simulink model "cesta"  (R2013a)
settings: Solver=ode3  StartTime=0.0  StopTime=10  FixedStep=0.01  RelTol=1e-3
values from neighbouring files (symbols this model uses):
  goalX = 900    [start.m]
  goalY = 900    [start.m]
  k1 = patch ([posx p1(1) p2(1) posx],[posy p1(2) p2(2) posy],'blue')    [start.m]    (also in viewMap.m = u(10))
  k2 = patch ([posx p2(1) p3(1) posx],[posy p2(2) p3(2) posy],'blue')    [start.m]    (also in viewMap.m = u(12))
  k3 = patch ([posx p3(1) p4(1) posx],[posy p3(2) p4(2) posy],'blue')    [start.m]    (also in viewMap.m = u(14))
  map = genRandMap(100,100,50)    [dummyTest.m]    (also in genRandMap.m = zeros(rows,columns); start.m)
  posx = 50    [start.m]
  posy = 50    [start.m]
  refAuto = patch([posx-xSize/2 posx+xSize/2 posx+xSize/2 posx-xSize/2], [posy-ySize/2 posy-ySize/2 posy+ySize/2 posy+ySize/2], 'green')    [start.m]    (also in viewMap.m = u(7))
  refK1 = patch ([posx p1(1) p2(1) posx],[posy p1(2) p2(2) posy],'blue')    [start.m]    (also in viewMap.m = u(9))
  refK2 = patch ([posx p2(1) p3(1) posx],[posy p2(2) p3(2) posy],'blue')    [start.m]    (also in viewMap.m = u(11))
  refK3 = patch ([posx p3(1) p4(1) posx],[posy p3(2) p4(2) posy],'blue')    [start.m]    (also in viewMap.m = u(13))
  sensRange = 100    [start.m]
undefined symbols (not defined in the file or in its folder): evalObstacles, viewMap
libraries: fuzblock x1
settings Model: Creator=Marek  LastModifiedBy=Marek

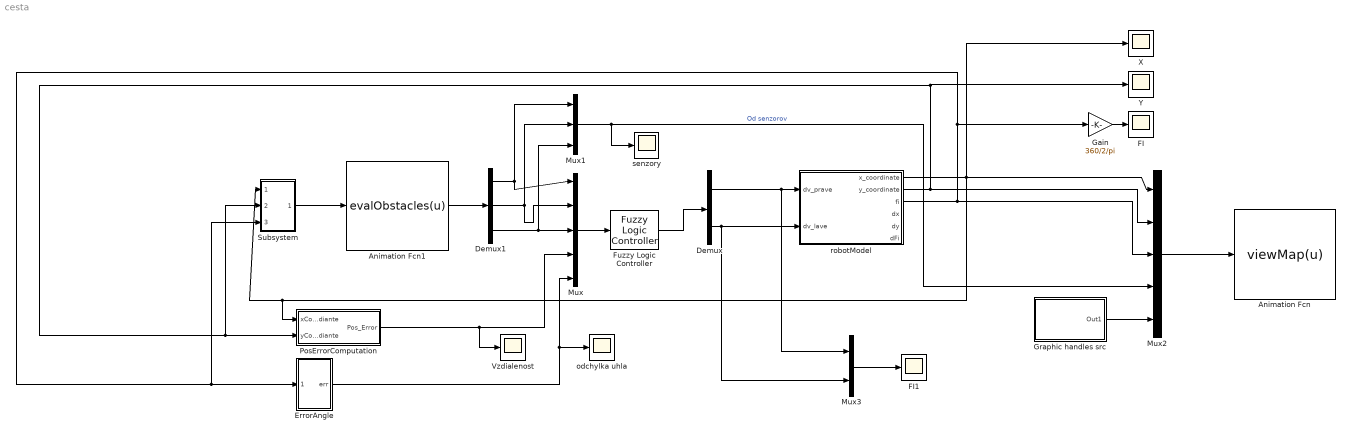
== system cesta ==
  Animation Fcn : MATLABFcn  MATLABFcn=viewMap(u)  OutputDimensions=0
  Animation Fcn1 : MATLABFcn  MATLABFcn=evalObstacles(u)  OutputDimensions=3
  Demux : Demux  Outputs=2
  Demux1 : Demux  Outputs=3
  ErrorAngle : Subsystem
  FI : Scope
      settings: YMin=0.564649  YMax=0.624085  SaveName=ScopeData5
  FI1 : Scope
      settings: YMin=33.51  YMax=33.5675  SaveName=ScopeData6
  Fuzzy Logic Controller : fuzblock/Fuzzy Logic  Controller  fis=fuzcar
  Gain : Gain  Gain=360/2/pi
  Graphic handles src : Subsystem
  Mux : Mux  Inputs=5
  Mux1 : Mux  Inputs=3
  Mux2 : Mux  Inputs=5
  Mux3 : Mux  Inputs=2
  PosErrorComputation : Subsystem
  Subsystem : Subsystem
  Vzdialenost : Scope
      settings: SaveName=ScopeData2
  X : Scope
      settings: YMin=45  YMax=90  SaveName=ScopeData11
  Y : Scope
      settings: YMin=32.4387  YMax=32.4417  SaveName=ScopeData12
  odchylka uhla : Scope
      settings: TimeRange=10  SaveName=ScopeData3
  robotModel : Subsystem
  senzory : Scope
      settings: SaveName=ScopeData4
  wires:
  Demux/1 -> Mux3/1, robotModel/1(dv_prave)
  robotModel/3("fi ") -> Mux2/3, Gain/1, Subsystem/3(Angle), ErrorAngle/1(angle)
  Mux2/1 -> Animation Fcn/1
  robotModel/2(y_coordinate) -> Mux2/2, Y/1, Subsystem/2(PosY), PosErrorComputation/2(yCoordiante)
  robotModel/1(x_coordinate) -> Subsystem/1(PosX), PosErrorComputation/1(xCoordiante), Mux2/1, X/1
  Mux/1 -> Fuzzy Logic Controller/1
  Demux1/1 -> Mux/1, Mux1/1
  Demux1/2 -> Mux/2, Mux1/2
  Demux1/3 -> Mux1/3, Mux/3
  PosErrorComputation/1(Pos_Error) -> Vzdialenost/1, Mux/4
  ErrorAngle/1(err) -> odchylka uhla/1, Mux/5
  Mux1/1 -> senzory/1, Mux2/4  "Od senzorov"
  Demux/2 -> robotModel/2(dv_lave), Mux3/2
  Fuzzy Logic Controller/1 -> Demux/1
  Graphic handles src/1(Out1) -> Mux2/5
  Gain/1 -> FI/1
  Mux3/1 -> FI1/1
  Animation Fcn1/1 -> Demux1/1
  Subsystem/1(Out1) -> Animation Fcn1/1

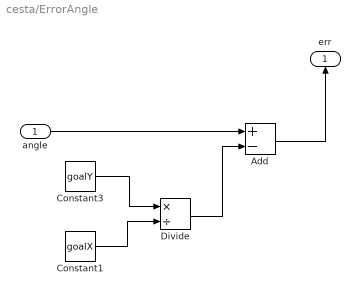
== system cesta/ErrorAngle ==
  angle : Inport
  Add : Sum  Inputs=+-
  Constant1 : Constant  Value=goalX
  Constant3 : Constant  Value=goalY
  Divide : Product  Inputs=*/
  err : Outport
  wires:
  Add/1 -> err/1
  Divide/1 -> Add/2
  angle/1 -> Add/1
  Constant3/1 -> Divide/1
  Constant1/1 -> Divide/2

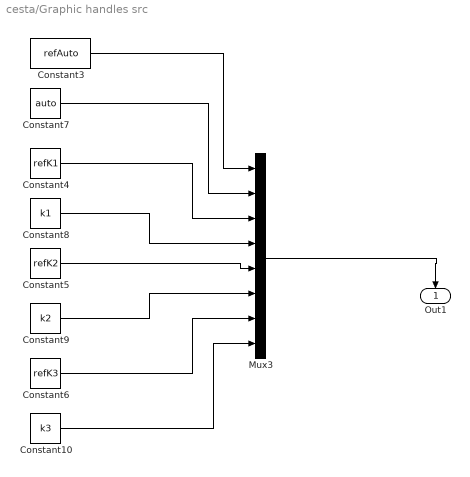
== system cesta/Graphic handles src ==
  Constant10 : Constant  Value=k3
  Constant3 : Constant  Value=refAuto
  Constant4 : Constant  Value=refK1
  Constant5 : Constant  Value=refK2
  Constant6 : Constant  Value=refK3
  Constant7 : Constant  Value=auto
  Constant8 : Constant  Value=k1
  Constant9 : Constant  Value=k2
  Mux3 : Mux  Inputs=8
  Out1 : Outport
  wires:
  Constant4/1 -> Mux3/3
  Mux3/1 -> Out1/1
  Constant6/1 -> Mux3/7
  Constant8/1 -> Mux3/4
  Constant9/1 -> Mux3/6
  Constant5/1 -> Mux3/5
  Constant10/1 -> Mux3/8
  Constant3/1 -> Mux3/1
  Constant7/1 -> Mux3/2

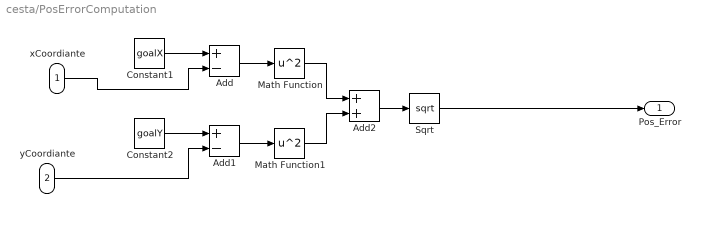
== system cesta/PosErrorComputation ==
  xCoordiante : Inport
  yCoordiante : Inport  Port=2
  Add : Sum  Inputs=+-
  Add1 : Sum  Inputs=+-
  Add2 : Sum
  Constant1 : Constant  Value=goalX
  Constant2 : Constant  Value=goalY
  Math Function : Math  Operator=square  SaturateOnIntegerOverflow=on
  Math Function1 : Math  Operator=square  SaturateOnIntegerOverflow=on
  Sqrt : Sqrt  SaturateOnIntegerOverflow=on
  Pos_Error : Outport
  wires:
  Add2/1 -> Sqrt/1
  Math Function/1 -> Add2/1
  Math Function1/1 -> Add2/2
  Constant2/1 -> Add1/1
  Add/1 -> Math Function/1
  Add1/1 -> Math Function1/1
  Constant1/1 -> Add/1
  Sqrt/1 -> Pos_Error/1
  xCoordiante/1 -> Add/2
  yCoordiante/1 -> Add1/2

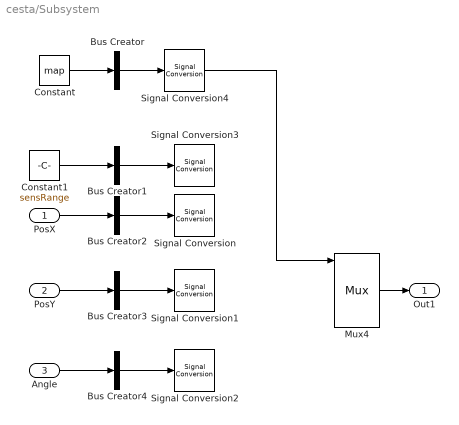
== system cesta/Subsystem ==
  PosX : Inport
  PosY : Inport  Port=2
  Angle : Inport  Port=3
  Bus Creator{,1..4} (5 alike) : BusCreator  Inputs=1
  Constant : Constant  Value=map  VectorParams1D=off
  Constant1 : Constant  Value=sensRange
  Mux4 : Mux  Inputs=5
  Signal Conversion{,1..4} (5 alike) : SignalConversion  ConversionOutput=Virtual bus
  Out1 : Outport
  wires:
  Mux4/1 -> Out1/1
  Signal Conversion4/1 -> Mux4/1
  Constant/1 -> Bus Creator/1
  Constant1/1 -> Bus Creator1/1
  PosX/1 -> Bus Creator2/1
  PosY/1 -> Bus Creator3/1
  Angle/1 -> Bus Creator4/1
  Bus Creator/1 -> Signal Conversion4/1
  Bus Creator1/1 -> Signal Conversion3/1
  Bus Creator2/1 -> Signal Conversion/1
  Bus Creator3/1 -> Signal Conversion1/1
  Bus Creator4/1 -> Signal Conversion2/1

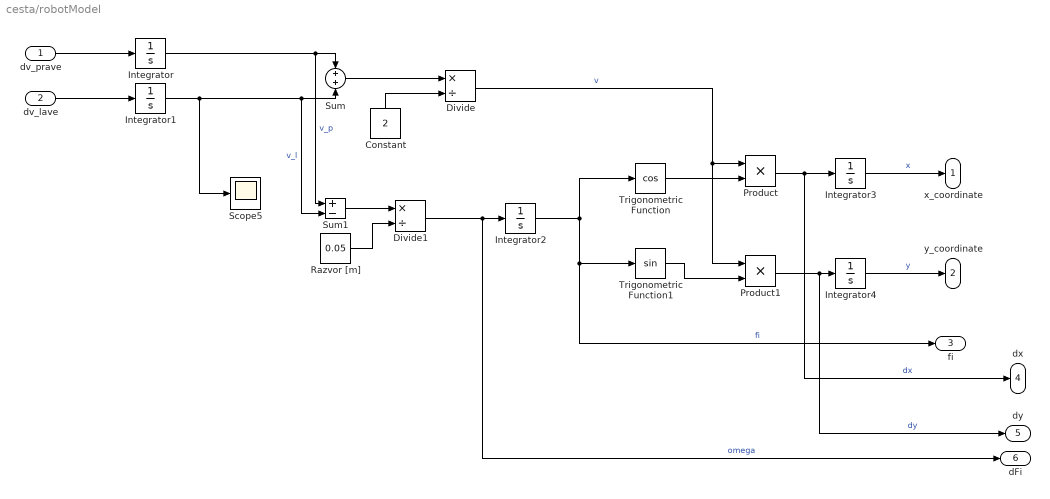
== system cesta/robotModel ==
  dv_prave : Inport
  dv_lave : Inport  Port=2
  Constant : Constant  Value=2
  Divide : Product  Inputs=*/
  Divide1 : Product  Inputs=*/
  Integrator : Integrator  LimitOutput=on  UpperSaturationLimit=20  LowerSaturationLimit=-20
  Integrator1 : Integrator  LimitOutput=on  UpperSaturationLimit=20  LowerSaturationLimit=-20
  Integrator2 : Integrator  InitialCondition=angle/360*2*pi
  Integrator3 : Integrator  InitialCondition=posx  UpperSaturationLimit=1000  LowerSaturationLimit=0
  Integrator4 : Integrator  InitialCondition=posy  UpperSaturationLimit=1000  LowerSaturationLimit=0
  Product : Product
  Product1 : Product
  Razvor [m] : Constant  Value=0.05
  Scope5 : Scope
      settings: YMin=32.4387  YMax=32.4417  SaveName=ScopeData8
  Sum : Sum
  Sum1 : Sum  Inputs=+-
  Trigonometric Function : Trigonometry  Operator=cos
  Trigonometric Function1 : Trigonometry
  x_coordinate : Outport
  y_coordinate : Outport  Port=2
  "fi " : Outport  Port=3
  dx : Outport  Port=4
  dy : Outport  Port=5
  dFi : Outport  Port=6
  wires:
  Divide/1 -> Product/1, Product1/1  "v"
  Integrator1/1 -> Scope5/1, Sum1/2, Sum/2  "v_l"
  Integrator/1 -> Sum1/1, Sum/1  "v_p"
  Constant/1 -> Divide/2
  Trigonometric Function/1 -> Product/2
  Integrator2/1 -> "fi "/1, Trigonometric Function1/1, Trigonometric Function/1  "fi"
  Product1/1 -> dy/1, Integrator4/1  "dy"
  Sum/1 -> Divide/1
  Product/1 -> dx/1, Integrator3/1  "dx"
  Trigonometric Function1/1 -> Product1/2
  dv_prave/1 -> Integrator/1
  dv_lave/1 -> Integrator1/1
  Sum1/1 -> Divide1/1
  Divide1/1 -> dFi/1, Integrator2/1  "omega"
  Razvor [m]/1 -> Divide1/2
  Integrator4/1 -> y_coordinate/1  "y"
  Integrator3/1 -> x_coordinate/1  "x"
